simulink model "line_CF1_FS"  (R2018b)
settings: Solver=FixedStepAuto  StartTime=0.0  StopTime=inf  FixedStep=0.01  RelTol=1e-3
undefined symbols (not defined in the file or in its folder): Angular, Linear
libraries: autolibshared x10, vehdynlibsteering x10, robotlib x7, peGeneralControl x1
(part 1 of 2)
settings Model: Creator=ckreienk  LastModifiedBy=ckreienk

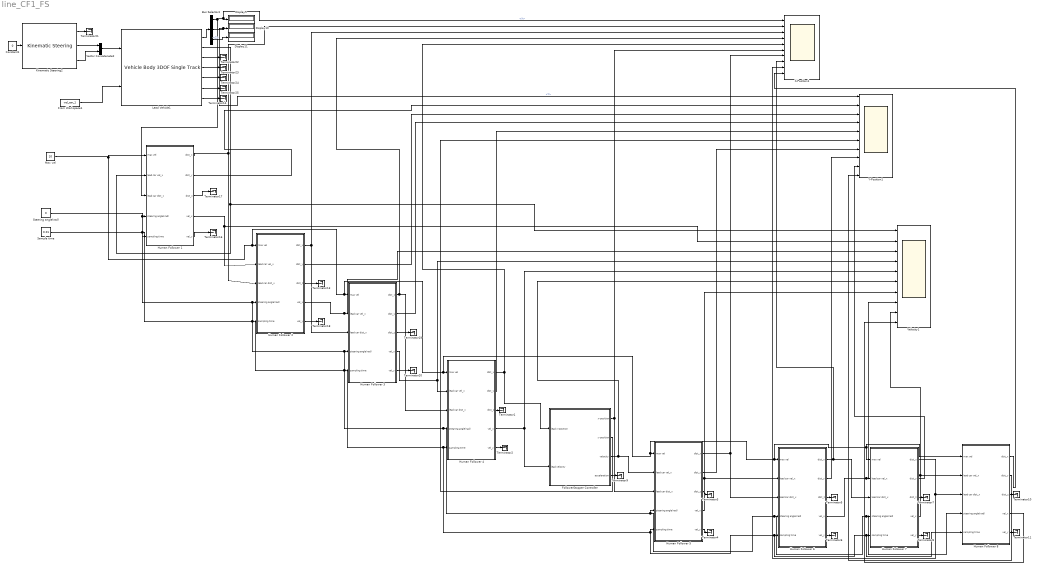
== system line_CF1_FS ==
  Bus Selector4 : BusSelector  OutputSignals=InertFrm.Geom.Disp.X,InertFrm.Geom.Disp.Y,InertFrm.Geom.Disp.Z
  Constant1 : Constant  Value=0
  Display10 : Display
  Display11 : Display
  Display9 : Display
  FollowerStopper Controller : Subsystem
  From Workspace1 : FromWorkspace  VariableName=vel_car_1  SampleTime=0.1
  Human Follower 1 : Subsystem
  Human Follower 2 : Subsystem
  Human Follower 3 : Subsystem
  Human Follower 4 : Subsystem
  Human Follower 5 : Subsystem
  Human Follower 6 : Subsystem
  Human Follower 7 : Subsystem
  Human Follower 8 : Subsystem
  Kinematic Steering2 : vehdynlibsteering/Kinematic Steering  StrgType=Rack and pinion  StrgRatioType=Constant  Loc=Front  NrmlFctr=0.01  TrckWdth=1  WhlBase=1.524  Db=0  StrgRng=1.25*pi  StrgAngBpts="[-6.2832   -5.0265   -3.7699   -2.5133   -1.2566         0    1.2566    2.5133    3.7699    5.0265    6.2832]"  StrgRatioTbl=|  StrgRatio=100  StrgArmLngth=0.1  RckCsLngth=0.5  TieRodLngth=0.248  D=0.2  PnnRadius=0.0057  PnnRadiusTbl="[0.0055    0.0055    0.0056    0.0057    0.0058    0.0057    0.0057    0.0057    0.0056    0.0055    0.0055]"  RodLngth=0.1  ParaArmLngth=0.9  aMode=2
      | [13.5000   13.3750   13.2500   13.1250   13.0000   13.0000   13.0000   13.1250   13.2500   13.3750   13.5000
      | ]
      settings: SourceProductName=Vehicle Dynamics Blockset
  Lead Vehicle1 : autolibshared/Vehicle Body 3DOF Single Track  trackMode=Dual  inputMode=External longitudinal velocity  frontSteerMode=on  rearSteerMode=off  windMode=off  muMode=off  extFMode=off  extMMode=off  aMode=2  NF=2  NR=2  m=2000  a=1.4  b=1.6  h=0.35  X_o=100  xdot_o=0  CalphaMode=off  sigmaMode=off  d=0  w=[1.4,1.4]  Cy_f=12e3  Cy_r=11e3  sigma_f=.1  sigma_r=.1  alpha_f_brk=[-.1 .1]  Cy_f_data=[-9e3 9e3]  alpha_r_brk=[-.1 .1]  Cy_r_data=[-9e3 9e3]  Y_o=0  ydot_o=0  Izz=4000  psi_o=0  r_o=0  Af=2  Cd=.3  Cl=.1  Cpm=.1  beta_w=[0:0.01:0.3]  Cs=[0:0.03:0.9]  Cym=[0:0.01:0.3]  Pabs=101325  Tair=273  g=9.81  mu=1  xdot_tol=.01  Fznom=5000  Fxtire_sat=7e4  Fytire_sat=7e4  longOff=0  latOff=0  vertOff=0
      settings: SourceProductName=Powertrain Blockset  SourceProductBaseCode=PW
  Max vel : Constant  Value=10
  Sample time : Constant  Value=0.01
  Steering angle(rad) : Constant  Value=0
  Terminator{1..11,13..14,16..25} (23 alike) : Terminator
  Vector Concatenate2 : Concatenate
  Velocity1 : Scope  NumInputPorts=10
  X-Position1 : Scope  NumInputPorts=10
  Y-Position1 : Scope  NumInputPorts=10
  wires:
  Human Follower 1/2(dist_y) -> Y-Position1/2
  Human Follower 2/5(vel_y) -> Terminator18/1
  Human Follower 1/4(vel_x) -> Human Follower 2/2(lead car vel_x), Velocity1/2
  Human Follower 3/5(vel_y) -> Terminator20/1
  Human Follower 3/4(vel_x) -> Human Follower 4/2(lead car vel_x), Velocity1/4
  Vector Concatenate2/1 -> Lead Vehicle1/1
  Lead Vehicle1/7 -> Terminator14/1
  Human Follower 1/1(dist_x) -> Human Follower 2/3(lead car dist_x), X-Position1/2
  Human Follower 2/1(dist_x) -> X-Position1/3, Human Follower 3/3(lead car dist_x)
  Sample time/1 -> Human Follower 8/5(sampling time), Human Follower 7/5(sampling time), Human Follower 6/5(sampling time), Human Follower 5/5(sampling time), Human Follower 4/5(sampling time), Human Follower 3/5(sampling time), Human Follower 2/5(sampling time), Human Follower 1/5(sampling time)
  Max vel/1 -> Human Follower 1/1(max vel), Human Follower 7/1(max vel), Human Follower 8/1(max vel), Human Follower 6/1(max vel), Human Follower 5/1(max vel), Human Follower 4/1(max vel), Human Follower 3/1(max vel), Human Follower 2/1(max vel)
  Lead Vehicle1/6 -> Terminator25/1
  Bus Selector4/1 -> Display9/1, X-Position1/1, Human Follower 1/3(lead car dist_x)  "<X>"
  Kinematic Steering2/2 -> Vector Concatenate2/1
  Lead Vehicle1/4 -> Terminator23/1
  Human Follower 1/3(dist_z) -> Terminator17/1
  Human Follower 2/4(vel_x) -> Velocity1/3, Human Follower 3/2(lead car vel_x)
  Lead Vehicle1/2 -> Human Follower 1/2(lead car vel_x), Velocity1/1
  Constant1/1 -> Kinematic Steering2/1
  Human Follower 2/3(dist_z) -> Terminator13/1
  Lead Vehicle1/1 -> Bus Selector4/1
  Lead Vehicle1/3 -> Terminator22/1
  Human Follower 3/3(dist_z) -> Terminator19/1
  From Workspace1/1 -> Lead Vehicle1/2
  Human Follower 2/2(dist_y) -> Y-Position1/3
  Human Follower 3/2(dist_y) -> Y-Position1/4
  Human Follower 3/1(dist_x) -> Human Follower 4/3(lead car dist_x), X-Position1/4
  Bus Selector4/2 -> Display10/1, Y-Position1/1  "<Y>"
  Kinematic Steering2/1 -> Terminator21/1
  Kinematic Steering2/3 -> Vector Concatenate2/2
  Bus Selector4/3 -> Display11/1  "<Z>"
  Human Follower 1/5(vel_y) -> Terminator16/1
  Lead Vehicle1/5 -> Terminator24/1
  Steering angle(rad)/1 -> Human Follower 8/4(stearing angle(rad)), Human Follower 7/4(stearing angle(rad)), Human Follower 6/4(stearing angle(rad)), Human Follower 5/4(stearing angle(rad)), Human Follower 4/4(stearing angle(rad)), Human Follower 3/4(stearing angle(rad)), Human Follower 2/4(stearing angle(rad)), Human Follower 1/4(stearing angle(rad))
  Human Follower 4/1(dist_x) -> X-Position1/5, FollowerStopper Controller/1(lead x-position)
  Human Follower 4/2(dist_y) -> Y-Position1/5
  Human Follower 4/3(dist_z) -> Terminator1/1
  Human Follower 4/5(vel_y) -> Terminator2/1
  Human Follower 4/4(vel_x) -> FollowerStopper Controller/2(lead velocity), Velocity1/5
  Human Follower 5/5(vel_y) -> Terminator4/1
  Human Follower 5/3(dist_z) -> Terminator3/1
  Human Follower 6/5(vel_y) -> Terminator6/1
  Human Follower 6/3(dist_z) -> Terminator5/1
  Human Follower 7/5(vel_y) -> Terminator8/1
  Human Follower 7/3(dist_z) -> Terminator7/1
  FollowerStopper Controller/1(x-position) -> Human Follower 5/3(lead car dist_x), X-Position1/6
  FollowerStopper Controller/2(y-position) -> Y-Position1/6
  FollowerStopper Controller/3(velocity) -> Human Follower 5/2(lead car vel_x), Velocity1/6
  FollowerStopper Controller/4(acceleration) -> Terminator9/1
  Human Follower 5/1(dist_x) -> Human Follower 6/3(lead car dist_x), X-Position1/7
  Human Follower 5/2(dist_y) -> Y-Position1/7
  Human Follower 5/4(vel_x) -> Human Follower 6/2(lead car vel_x), Velocity1/7
  Human Follower 6/1(dist_x) -> X-Position1/8, Human Follower 7/3(lead car dist_x)
  Human Follower 6/2(dist_y) -> Y-Position1/8
  Human Follower 6/4(vel_x) -> Velocity1/8, Human Follower 7/2(lead car vel_x)
  Human Follower 7/4(vel_x) -> Velocity1/9, Human Follower 8/2(lead car vel_x)
  Human Follower 7/2(dist_y) -> Y-Position1/9
  Human Follower 7/1(dist_x) -> Human Follower 8/3(lead car dist_x), X-Position1/9
  Human Follower 8/1(dist_x) -> X-Position1/10
  Human Follower 8/2(dist_y) -> Y-Position1/10
  Human Follower 8/3(dist_z) -> Terminator10/1
  Human Follower 8/5(vel_y) -> Terminator11/1
  Human Follower 8/4(vel_x) -> Velocity1/10

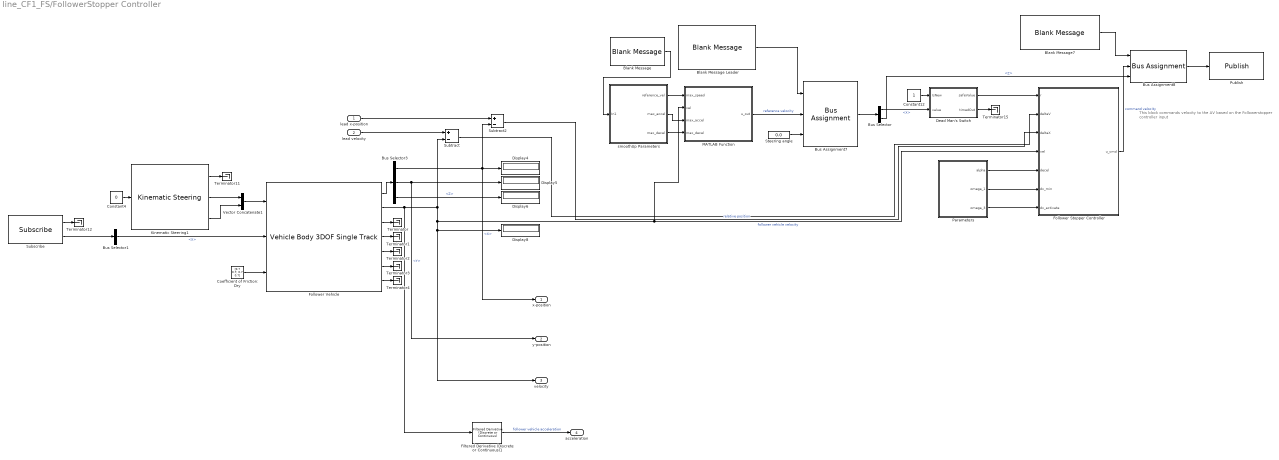
== system line_CF1_FS/FollowerStopper Controller ==
  note: This block commands velocity to the AV based
      | on the Followerstopper controller input
  lead x-position : Inport
  lead velocity : Inport  Port=2
  Blank Message : robotlib/Blank Message  messageClass=Message  entityType=geometry_msgs/Point  messageType=geometry_msgs/Point  SampleTime=inf
      settings: SourceProductBaseCode=RO
  Blank Message Leader : robotlib/Blank Message  messageClass=Message  entityType=geometry_msgs/Twist  messageType=geometry_msgs/Twist  SampleTime=inf
      settings: SourceProductBaseCode=RO
  Blank Message7 : robotlib/Blank Message  messageClass=Message  entityType=geometry_msgs/Twist  messageType=geometry_msgs/Twist  SampleTime=inf
      settings: SourceProductBaseCode=RO
  Bus Assignment7 : BusAssignment  AssignedSignals=Linear.X,Angular.Z
  Bus Assignment8 : BusAssignment  AssignedSignals=Linear.X,Angular.Z
  Bus Selector : BusSelector  OutputSignals=Linear.X,Angular.Z
  Bus Selector1 : BusSelector  OutputSignals=Linear.X
  Bus Selector3 : BusSelector  OutputSignals=InertFrm.Geom.Disp.X,InertFrm.Geom.Disp.Y,InertFrm.Geom.Disp.Z
  Coefficient of Friction: Dry : Constant  Value=[0.7 0.7; 0.7 0.7]
  Constant12 : Constant
  Constant4 : Constant  Value=0
  Dead Man's Switch : Subsystem  TreatAsAtomicUnit=on  mask{stepSize=0.05, timeout=0.2}
      mask prompts: stepSize "Simulation step size"; timeout "Timeout (in seconds)"
      mask help: Interprets whether a new message has been recently received, and if so permits the data in 'value' to be passed through. Otherwise, 0 is outputted from 'safeValue'
      mask Help: Interprets whether a new message has been recently received, and if so permits the data in 'value' to be passed through. Otherwise, 0 is outputted from 'safeValue'
  Display{4..6,8} (4 alike) : Display
  Filtered Derivative (Discrete or Continuous)1 : peGeneralControl/Filtered Derivative (Discrete or Continuous)  K=1  T=0.1  B=20  A=-20  minRatio=10  Ts=-1
  Follower Stopper Controller : Subsystem
  Follower Vehicle : autolibshared/Vehicle Body 3DOF Single Track  trackMode=Dual  inputMode=External longitudinal velocity  frontSteerMode=on  rearSteerMode=off  windMode=off  muMode=on  extFMode=off  extMMode=off  aMode=2  NF=2  NR=2  m=2000  a=1.4  b=1.6  h=0.35  X_o=50  xdot_o=0  CalphaMode=off  sigmaMode=on  d=0  w=[1.4,1.4]  Cy_f=12e3  Cy_r=11e3  sigma_f=.1  sigma_r=.1  alpha_f_brk=[-.1 .1]  Cy_f_data=[-9e3 9e3]  alpha_r_brk=[-.1 .1]  Cy_r_data=[-9e3 9e3]  Y_o=0  ydot_o=0  Izz=4000  psi_o=0  r_o=0  Af=2  Cd=.3  Cl=.1  Cpm=.1  beta_w=[0:0.01:0.3]  Cs=[0:0.03:0.9]  Cym=[0:0.01:0.3]  Pabs=101325  Tair=273  g=9.81  mu=1  xdot_tol=.01  Fznom=5000  Fxtire_sat=7e4  Fytire_sat=7e4  longOff=0  latOff=0  vertOff=0
      settings: SourceProductName=Powertrain Blockset  SourceProductBaseCode=PW
  Kinematic Steering1 : vehdynlibsteering/Kinematic Steering  StrgType=Rack and pinion  StrgRatioType=Constant  Loc=Front  NrmlFctr=0.01  TrckWdth=1  WhlBase=1.524  Db=0  StrgRng=1.25*pi  StrgAngBpts="[-6.2832   -5.0265   -3.7699   -2.5133   -1.2566         0    1.2566    2.5133    3.7699    5.0265    6.2832]"  StrgRatioTbl=|  StrgRatio=100  StrgArmLngth=0.1  RckCsLngth=0.5  TieRodLngth=0.248  D=0.2  PnnRadius=0.0057  PnnRadiusTbl="[0.0055    0.0055    0.0056    0.0057    0.0058    0.0057    0.0057    0.0057    0.0056    0.0055    0.0055]"  RodLngth=0.1  ParaArmLngth=0.9  aMode=2
      | [13.5000   13.3750   13.2500   13.1250   13.0000   13.0000   13.0000   13.1250   13.2500   13.3750   13.5000
      | ]
      settings: SourceProductName=Vehicle Dynamics Blockset
  MATLAB Function : MATLAB Function  TreatAsAtomicUnit=on
  Parameters : Subsystem
  Publish : robotlib/Publish  topicSource=Specify your own  topic=cmd_vel  messageType=geometry_msgs/Twist  messageQueueLength=1
      settings: SourceProductBaseCode=RO
  Steering angle : Constant  Value=0.0
  Subscribe : robotlib/Subscribe  topicSource=Specify your own  topic=cmd_vel  messageType=geometry_msgs/Twist  sampleTime=-1  messageQueueLength=1
      settings: SourceProductBaseCode=RO
  Subtract : Sum  Inputs=+-
  Subtract2 : Sum  Inputs=+-
  Terminator{,1..4,11..12,15} (8 alike) : Terminator
  Vector Concatenate1 : Concatenate
  smoothUp Parameters : Subsystem
  x-position : Outport
  y-position : Outport  Port=2
  velocity : Outport  Port=3
  acceleration : Outport  Port=4
  wires:
  Follower Vehicle/7 -> Terminator4/1
  MATLAB Function/1(u_out) -> Bus Assignment7/2  "reference velocity"
  Constant4/1 -> Kinematic Steering1/1
  Parameters/3(omega_3) -> Follower Stopper Controller/7(dx_activate)
  Bus Selector3/2 -> y-position/1, Display5/1  "<Y>"
  Steering angle/1 -> Bus Assignment7/3
  Follower Vehicle/5 -> Terminator2/1
  Constant12/1 -> Dead Man's Switch/1(IsNew)
  Subtract2/1 -> Follower Stopper Controller/3(deltaX)  "relative position"
  Dead Man's Switch/1(safeValue) -> Follower Stopper Controller/1(r)
  Kinematic Steering1/1 -> Terminator11/1
  Bus Selector/1 -> Dead Man's Switch/2(value)  "<X>"
  Bus Selector3/3 -> Display6/1  "<Z>"
  Dead Man's Switch/2(timedOut) -> Terminator15/1
  Subscribe/1 -> Terminator12/1
  Follower Vehicle/2 -> Filtered Derivative (Discrete or Continuous)1/1, velocity/1, Display8/1, MATLAB Function/2(vel), Follower Stopper Controller/4(vel), Subtract/2  "follower vehicle velocity"
  lead x-position/1 -> Subtract2/1
  Parameters/2(omega_1) -> Follower Stopper Controller/6(dx_min)
  Follower Stopper Controller/1(u_cmd) -> Bus Assignment8/2  "command velocity"
  Bus Selector3/1 -> x-position/1, Display4/1, Subtract2/2  "<X>"
  Blank Message/1 -> smoothUp Parameters/1(In1)
  Bus Selector1/1 -> Follower Vehicle/2  "<X>"
  Vector Concatenate1/1 -> Follower Vehicle/1
  Subtract/1 -> Follower Stopper Controller/2(deltaV)
  Blank Message Leader/1 -> Bus Assignment7/1
  Filtered Derivative (Discrete or Continuous)1/1 -> acceleration/1  "follower vehicle acceleration"
  Bus Selector/2 -> Bus Assignment8/3  "<Z>"
  Bus Assignment8/1 -> Publish/1
  Bus Assignment7/1 -> Bus Selector/1
  smoothUp Parameters/1(reference_vel) -> MATLAB Function/1(max_speed)
  Coefficient of Friction: Dry/1 -> Follower Vehicle/3
  Follower Vehicle/6 -> Terminator3/1
  Blank Message7/1 -> Bus Assignment8/1
  smoothUp Parameters/2(max_accel) -> MATLAB Function/3(max_accel)
  Follower Vehicle/1 -> Bus Selector3/1
  Follower Vehicle/3 -> Terminator/1
  Kinematic Steering1/2 -> Vector Concatenate1/1
  Kinematic Steering1/3 -> Vector Concatenate1/2
  Subscribe/2 -> Bus Selector1/1
  Parameters/1(alpha) -> Follower Stopper Controller/5(decel)
  lead velocity/1 -> Subtract/1
  smoothUp Parameters/3(max_decel) -> MATLAB Function/4(max_decel)
  Follower Vehicle/4 -> Terminator1/1

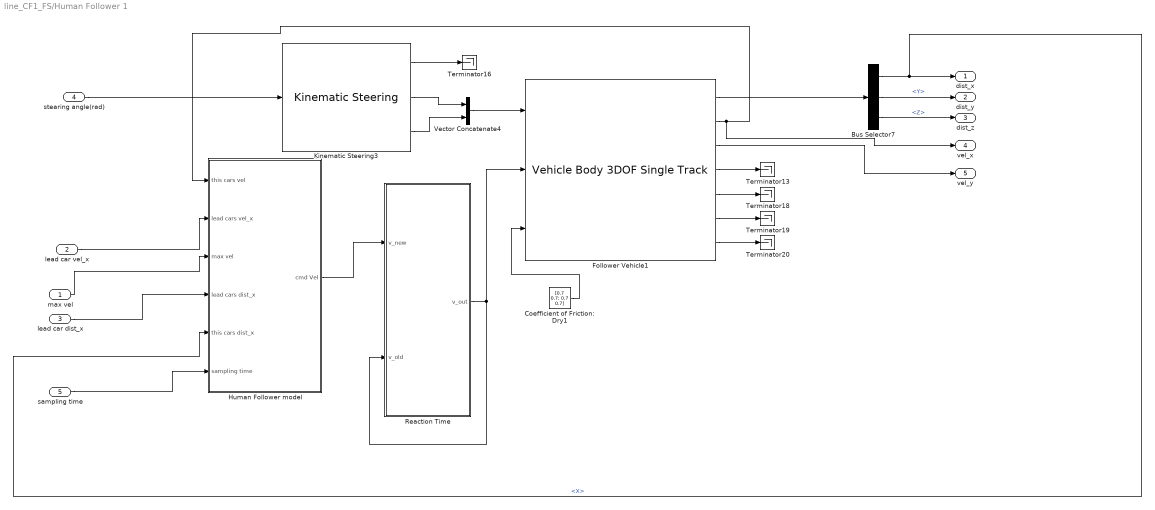
== system line_CF1_FS/Human Follower 1 ==
  max vel : Inport
  lead car vel_x : Inport  Port=2
  lead car dist_x : Inport  Port=3
  stearing angle(rad) : Inport  Port=4
  sampling time : Inport  Port=5
  Bus Selector7 : BusSelector  OutputSignals=InertFrm.Cg.Disp.X,InertFrm.Cg.Disp.Y,InertFrm.Cg.Disp.Z
  Coefficient of Friction: Dry1 : Constant  Value=[0.7 0.7; 0.7 0.7]
  Follower Vehicle1 : autolibshared/Vehicle Body 3DOF Single Track  trackMode=Dual  inputMode=External longitudinal velocity  frontSteerMode=on  rearSteerMode=off  windMode=off  muMode=on  extFMode=off  extMMode=off  aMode=2  NF=2  NR=2  m=2000  a=1.4  b=1.6  h=0.35  X_o=90  xdot_o=0  CalphaMode=off  sigmaMode=on  d=0  w=[1.4,1.4]  Cy_f=12e3  Cy_r=11e3  sigma_f=.1  sigma_r=.1  alpha_f_brk=[-.1 .1]  Cy_f_data=[-9e3 9e3]  alpha_r_brk=[-.1 .1]  Cy_r_data=[-9e3 9e3]  Y_o=0  ydot_o=0  Izz=4000  psi_o=0  r_o=0  Af=2  Cd=.3  Cl=.1  Cpm=.1  beta_w=[0:0.01:0.3]  Cs=[0:0.03:0.9]  Cym=[0:0.01:0.3]  Pabs=101325  Tair=273  g=9.81  mu=1  xdot_tol=.01  Fznom=5000  Fxtire_sat=7e4  Fytire_sat=7e4  longOff=0  latOff=0  vertOff=0
      settings: SourceProductName=Powertrain Blockset  SourceProductBaseCode=PW
  Human Follower model : Subsystem
  Kinematic Steering3 : vehdynlibsteering/Kinematic Steering  StrgType=Rack and pinion  StrgRatioType=Constant  Loc=Front  NrmlFctr=0.01  TrckWdth=1  WhlBase=1.524  Db=0  StrgRng=1.25*pi  StrgAngBpts="[-6.2832   -5.0265   -3.7699   -2.5133   -1.2566         0    1.2566    2.5133    3.7699    5.0265    6.2832]"  StrgRatioTbl=|  StrgRatio=100  StrgArmLngth=0.1  RckCsLngth=0.5  TieRodLngth=0.248  D=0.2  PnnRadius=0.0057  PnnRadiusTbl="[0.0055    0.0055    0.0056    0.0057    0.0058    0.0057    0.0057    0.0057    0.0056    0.0055    0.0055]"  RodLngth=0.1  ParaArmLngth=0.9  aMode=2
      | [13.5000   13.3750   13.2500   13.1250   13.0000   13.0000   13.0000   13.1250   13.2500   13.3750   13.5000
      | ]
      settings: SourceProductName=Vehicle Dynamics Blockset
  Reaction Time : Subsystem
  Terminator{13,16,18..20} (5 alike) : Terminator
  Vector Concatenate4 : Concatenate
  dist_x : Outport
  dist_y : Outport  Port=2
  dist_z : Outport  Port=3
  vel_x : Outport  Port=4
  vel_y : Outport  Port=5
  wires:
  Bus Selector7/3 -> dist_z/1  "<Z>"
  Follower Vehicle1/5 -> Terminator18/1
  max vel/1 -> Human Follower model/3(max vel)
  Follower Vehicle1/6 -> Terminator19/1
  Bus Selector7/1 -> dist_x/1, Human Follower model/5(this cars dist_x)  "<X>"
  Follower Vehicle1/4 -> Terminator13/1
  Follower Vehicle1/3 -> vel_y/1
  lead car vel_x/1 -> Human Follower model/2(lead cars vel_x)
  Follower Vehicle1/7 -> Terminator20/1
  Vector Concatenate4/1 -> Follower Vehicle1/1
  Follower Vehicle1/1 -> Bus Selector7/1
  Kinematic Steering3/1 -> Terminator16/1
  lead car dist_x/1 -> Human Follower model/4(lead cars dist_x)
  Bus Selector7/2 -> dist_y/1  "<Y>"
  Kinematic Steering3/2 -> Vector Concatenate4/1
  stearing angle(rad)/1 -> Kinematic Steering3/1
  Kinematic Steering3/3 -> Vector Concatenate4/2
  Follower Vehicle1/2 -> Human Follower model/1(this cars vel), vel_x/1
  Coefficient of Friction: Dry1/1 -> Follower Vehicle1/3
  sampling time/1 -> Human Follower model/6(sampling time)
  Reaction Time/1(v_out) -> Follower Vehicle1/2, Reaction Time/2(v_old)
  Human Follower model/1(cmd Vel) -> Reaction Time/1(v_new)

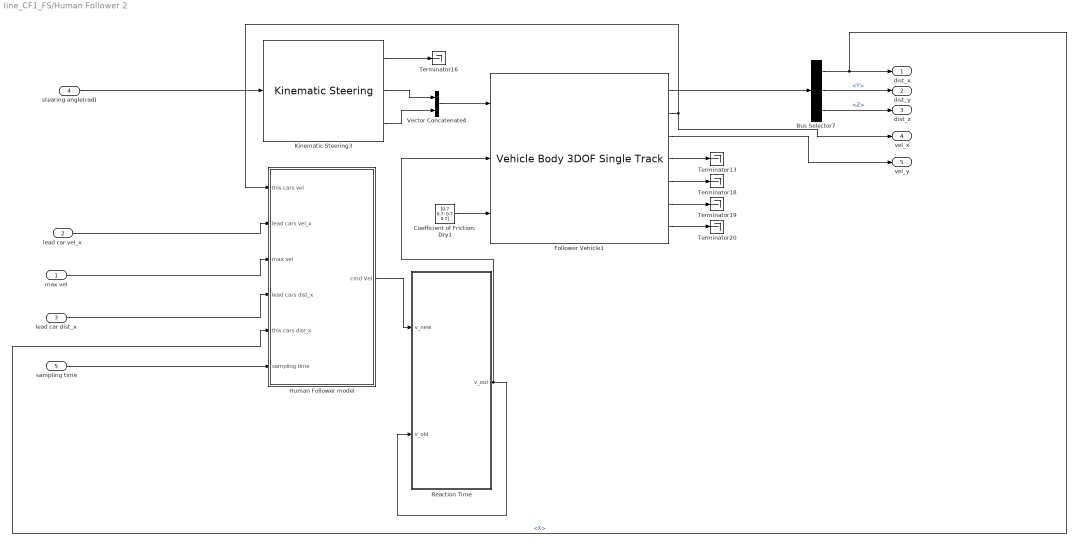
== system line_CF1_FS/Human Follower 2 ==
  max vel : Inport
  lead car vel_x : Inport  Port=2
  lead car dist_x : Inport  Port=3
  stearing angle(rad) : Inport  Port=4
  sampling time : Inport  Port=5
  Bus Selector7 : BusSelector  OutputSignals=InertFrm.Cg.Disp.X,InertFrm.Cg.Disp.Y,InertFrm.Cg.Disp.Z
  Coefficient of Friction: Dry1 : Constant  Value=[0.7 0.7; 0.7 0.7]
  Follower Vehicle1 : autolibshared/Vehicle Body 3DOF Single Track  trackMode=Dual  inputMode=External longitudinal velocity  frontSteerMode=on  rearSteerMode=off  windMode=off  muMode=on  extFMode=off  extMMode=off  aMode=2  NF=2  NR=2  m=2000  a=1.4  b=1.6  h=0.35  X_o=80  xdot_o=0  CalphaMode=off  sigmaMode=on  d=0  w=[1.4,1.4]  Cy_f=12e3  Cy_r=11e3  sigma_f=.1  sigma_r=.1  alpha_f_brk=[-.1 .1]  Cy_f_data=[-9e3 9e3]  alpha_r_brk=[-.1 .1]  Cy_r_data=[-9e3 9e3]  Y_o=0  ydot_o=0  Izz=4000  psi_o=0  r_o=0  Af=2  Cd=.3  Cl=.1  Cpm=.1  beta_w=[0:0.01:0.3]  Cs=[0:0.03:0.9]  Cym=[0:0.01:0.3]  Pabs=101325  Tair=273  g=9.81  mu=1  xdot_tol=.01  Fznom=5000  Fxtire_sat=7e4  Fytire_sat=7e4  longOff=0  latOff=0  vertOff=0
      settings: SourceProductName=Powertrain Blockset  SourceProductBaseCode=PW
  Human Follower model : Subsystem
  Kinematic Steering3 : vehdynlibsteering/Kinematic Steering  StrgType=Rack and pinion  StrgRatioType=Constant  Loc=Front  NrmlFctr=0.01  TrckWdth=1  WhlBase=1.524  Db=0  StrgRng=1.25*pi  StrgAngBpts="[-6.2832   -5.0265   -3.7699   -2.5133   -1.2566         0    1.2566    2.5133    3.7699    5.0265    6.2832]"  StrgRatioTbl=|  StrgRatio=100  StrgArmLngth=0.1  RckCsLngth=0.5  TieRodLngth=0.248  D=0.2  PnnRadius=0.0057  PnnRadiusTbl="[0.0055    0.0055    0.0056    0.0057    0.0058    0.0057    0.0057    0.0057    0.0056    0.0055    0.0055]"  RodLngth=0.1  ParaArmLngth=0.9  aMode=2
      | [13.5000   13.3750   13.2500   13.1250   13.0000   13.0000   13.0000   13.1250   13.2500   13.3750   13.5000
      | ]
      settings: SourceProductName=Vehicle Dynamics Blockset
  Reaction Time : Subsystem
  Terminator{13,16,18..20} (5 alike) : Terminator
  Vector Concatenate4 : Concatenate
  dist_x : Outport
  dist_y : Outport  Port=2
  dist_z : Outport  Port=3
  vel_x : Outport  Port=4
  vel_y : Outport  Port=5
  wires:
  Bus Selector7/3 -> dist_z/1  "<Z>"
  Follower Vehicle1/5 -> Terminator18/1
  max vel/1 -> Human Follower model/3(max vel)
  Follower Vehicle1/6 -> Terminator19/1
  Bus Selector7/1 -> dist_x/1, Human Follower model/5(this cars dist_x)  "<X>"
  Follower Vehicle1/4 -> Terminator13/1
  Follower Vehicle1/3 -> vel_y/1
  lead car vel_x/1 -> Human Follower model/2(lead cars vel_x)
  Follower Vehicle1/7 -> Terminator20/1
  Vector Concatenate4/1 -> Follower Vehicle1/1
  Follower Vehicle1/1 -> Bus Selector7/1
  Kinematic Steering3/1 -> Terminator16/1
  lead car dist_x/1 -> Human Follower model/4(lead cars dist_x)
  Bus Selector7/2 -> dist_y/1  "<Y>"
  sampling time/1 -> Human Follower model/6(sampling time)
  Kinematic Steering3/2 -> Vector Concatenate4/1
  stearing angle(rad)/1 -> Kinematic Steering3/1
  Kinematic Steering3/3 -> Vector Concatenate4/2
  Follower Vehicle1/2 -> Human Follower model/1(this cars vel), vel_x/1
  Coefficient of Friction: Dry1/1 -> Follower Vehicle1/3
  Reaction Time/1(v_out) -> Follower Vehicle1/2, Reaction Time/2(v_old)
  Human Follower model/1(cmd Vel) -> Reaction Time/1(v_new)

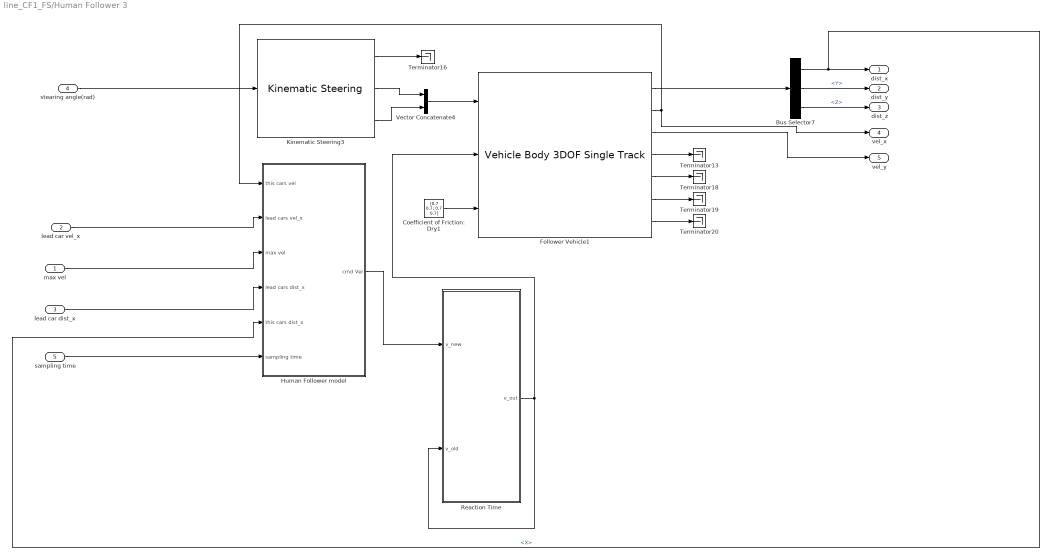
== system line_CF1_FS/Human Follower 3 ==
  max vel : Inport
  lead car vel_x : Inport  Port=2
  lead car dist_x : Inport  Port=3
  stearing angle(rad) : Inport  Port=4
  sampling time : Inport  Port=5
  Bus Selector7 : BusSelector  OutputSignals=InertFrm.Cg.Disp.X,InertFrm.Cg.Disp.Y,InertFrm.Cg.Disp.Z
  Coefficient of Friction: Dry1 : Constant  Value=[0.7 0.7; 0.7 0.7]
  Follower Vehicle1 : autolibshared/Vehicle Body 3DOF Single Track  trackMode=Dual  inputMode=External longitudinal velocity  frontSteerMode=on  rearSteerMode=off  windMode=off  muMode=on  extFMode=off  extMMode=off  aMode=2  NF=2  NR=2  m=2000  a=1.4  b=1.6  h=0.35  X_o=70  xdot_o=0  CalphaMode=off  sigmaMode=on  d=0  w=[1.4,1.4]  Cy_f=12e3  Cy_r=11e3  sigma_f=.1  sigma_r=.1  alpha_f_brk=[-.1 .1]  Cy_f_data=[-9e3 9e3]  alpha_r_brk=[-.1 .1]  Cy_r_data=[-9e3 9e3]  Y_o=0  ydot_o=0  Izz=4000  psi_o=0  r_o=0  Af=2  Cd=.3  Cl=.1  Cpm=.1  beta_w=[0:0.01:0.3]  Cs=[0:0.03:0.9]  Cym=[0:0.01:0.3]  Pabs=101325  Tair=273  g=9.81  mu=1  xdot_tol=.01  Fznom=5000  Fxtire_sat=7e4  Fytire_sat=7e4  longOff=0  latOff=0  vertOff=0
      settings: SourceProductName=Powertrain Blockset  SourceProductBaseCode=PW
  Human Follower model : Subsystem
  Kinematic Steering3 : vehdynlibsteering/Kinematic Steering  StrgType=Rack and pinion  StrgRatioType=Constant  Loc=Front  NrmlFctr=0.01  TrckWdth=1  WhlBase=1.524  Db=0  StrgRng=1.25*pi  StrgAngBpts="[-6.2832   -5.0265   -3.7699   -2.5133   -1.2566         0    1.2566    2.5133    3.7699    5.0265    6.2832]"  StrgRatioTbl=|  StrgRatio=100  StrgArmLngth=0.1  RckCsLngth=0.5  TieRodLngth=0.248  D=0.2  PnnRadius=0.0057  PnnRadiusTbl="[0.0055    0.0055    0.0056    0.0057    0.0058    0.0057    0.0057    0.0057    0.0056    0.0055    0.0055]"  RodLngth=0.1  ParaArmLngth=0.9  aMode=2
      | [13.5000   13.3750   13.2500   13.1250   13.0000   13.0000   13.0000   13.1250   13.2500   13.3750   13.5000
      | ]
      settings: SourceProductName=Vehicle Dynamics Blockset
  Reaction Time : Subsystem
  Terminator{13,16,18..20} (5 alike) : Terminator
  Vector Concatenate4 : Concatenate
  dist_x : Outport
  dist_y : Outport  Port=2
  dist_z : Outport  Port=3
  vel_x : Outport  Port=4
  vel_y : Outport  Port=5
  wires:
  Bus Selector7/3 -> dist_z/1  "<Z>"
  Follower Vehicle1/5 -> Terminator18/1
  max vel/1 -> Human Follower model/3(max vel)
  Follower Vehicle1/6 -> Terminator19/1
  Bus Selector7/1 -> dist_x/1, Human Follower model/5(this cars dist_x)  "<X>"
  Follower Vehicle1/4 -> Terminator13/1
  Follower Vehicle1/3 -> vel_y/1
  lead car vel_x/1 -> Human Follower model/2(lead cars vel_x)
  Follower Vehicle1/7 -> Terminator20/1
  Vector Concatenate4/1 -> Follower Vehicle1/1
  Follower Vehicle1/1 -> Bus Selector7/1
  Kinematic Steering3/1 -> Terminator16/1
  lead car dist_x/1 -> Human Follower model/4(lead cars dist_x)
  Bus Selector7/2 -> dist_y/1  "<Y>"
  sampling time/1 -> Human Follower model/6(sampling time)
  Kinematic Steering3/2 -> Vector Concatenate4/1
  stearing angle(rad)/1 -> Kinematic Steering3/1
  Kinematic Steering3/3 -> Vector Concatenate4/2
  Follower Vehicle1/2 -> Human Follower model/1(this cars vel), vel_x/1
  Coefficient of Friction: Dry1/1 -> Follower Vehicle1/3
  Reaction Time/1(v_out) -> Follower Vehicle1/2, Reaction Time/2(v_old)
  Human Follower model/1(cmd Vel) -> Reaction Time/1(v_new)

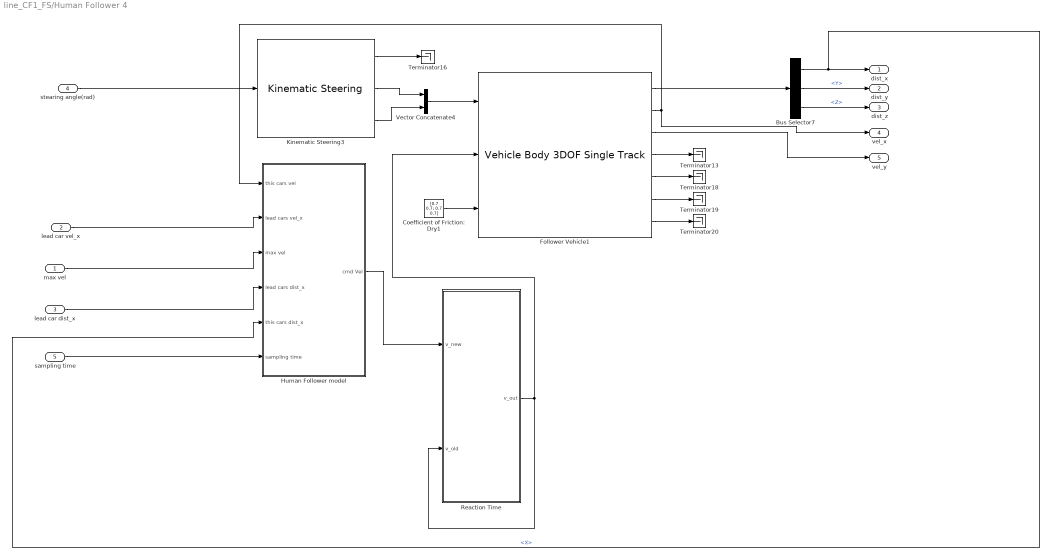
== system line_CF1_FS/Human Follower 4 ==
  max vel : Inport
  lead car vel_x : Inport  Port=2
  lead car dist_x : Inport  Port=3
  stearing angle(rad) : Inport  Port=4
  sampling time : Inport  Port=5
  Bus Selector7 : BusSelector  OutputSignals=InertFrm.Cg.Disp.X,InertFrm.Cg.Disp.Y,InertFrm.Cg.Disp.Z
  Coefficient of Friction: Dry1 : Constant  Value=[0.7 0.7; 0.7 0.7]
  Follower Vehicle1 : autolibshared/Vehicle Body 3DOF Single Track  trackMode=Dual  inputMode=External longitudinal velocity  frontSteerMode=on  rearSteerMode=off  windMode=off  muMode=on  extFMode=off  extMMode=off  aMode=2  NF=2  NR=2  m=2000  a=1.4  b=1.6  h=0.35  X_o=60  xdot_o=0  CalphaMode=off  sigmaMode=on  d=0  w=[1.4,1.4]  Cy_f=12e3  Cy_r=11e3  sigma_f=.1  sigma_r=.1  alpha_f_brk=[-.1 .1]  Cy_f_data=[-9e3 9e3]  alpha_r_brk=[-.1 .1]  Cy_r_data=[-9e3 9e3]  Y_o=0  ydot_o=0  Izz=4000  psi_o=0  r_o=0  Af=2  Cd=.3  Cl=.1  Cpm=.1  beta_w=[0:0.01:0.3]  Cs=[0:0.03:0.9]  Cym=[0:0.01:0.3]  Pabs=101325  Tair=273  g=9.81  mu=1  xdot_tol=.01  Fznom=5000  Fxtire_sat=7e4  Fytire_sat=7e4  longOff=0  latOff=0  vertOff=0
      settings: SourceProductName=Powertrain Blockset  SourceProductBaseCode=PW
  Human Follower model : Subsystem
  Kinematic Steering3 : vehdynlibsteering/Kinematic Steering  StrgType=Rack and pinion  StrgRatioType=Constant  Loc=Front  NrmlFctr=0.01  TrckWdth=1  WhlBase=1.524  Db=0  StrgRng=1.25*pi  StrgAngBpts="[-6.2832   -5.0265   -3.7699   -2.5133   -1.2566         0    1.2566    2.5133    3.7699    5.0265    6.2832]"  StrgRatioTbl=|  StrgRatio=100  StrgArmLngth=0.1  RckCsLngth=0.5  TieRodLngth=0.248  D=0.2  PnnRadius=0.0057  PnnRadiusTbl="[0.0055    0.0055    0.0056    0.0057    0.0058    0.0057    0.0057    0.0057    0.0056    0.0055    0.0055]"  RodLngth=0.1  ParaArmLngth=0.9  aMode=2
      | [13.5000   13.3750   13.2500   13.1250   13.0000   13.0000   13.0000   13.1250   13.2500   13.3750   13.5000
      | ]
      settings: SourceProductName=Vehicle Dynamics Blockset
  Reaction Time : Subsystem
  Terminator{13,16,18..20} (5 alike) : Terminator
  Vector Concatenate4 : Concatenate
  dist_x : Outport
  dist_y : Outport  Port=2
  dist_z : Outport  Port=3
  vel_x : Outport  Port=4
  vel_y : Outport  Port=5
  wires:
  Bus Selector7/3 -> dist_z/1  "<Z>"
  Follower Vehicle1/5 -> Terminator18/1
  max vel/1 -> Human Follower model/3(max vel)
  Follower Vehicle1/6 -> Terminator19/1
  Bus Selector7/1 -> dist_x/1, Human Follower model/5(this cars dist_x)  "<X>"
  Follower Vehicle1/4 -> Terminator13/1
  Follower Vehicle1/3 -> vel_y/1
  lead car vel_x/1 -> Human Follower model/2(lead cars vel_x)
  Follower Vehicle1/7 -> Terminator20/1
  Vector Concatenate4/1 -> Follower Vehicle1/1
  Follower Vehicle1/1 -> Bus Selector7/1
  Kinematic Steering3/1 -> Terminator16/1
  lead car dist_x/1 -> Human Follower model/4(lead cars dist_x)
  Bus Selector7/2 -> dist_y/1  "<Y>"
  sampling time/1 -> Human Follower model/6(sampling time)
  Kinematic Steering3/2 -> Vector Concatenate4/1
  stearing angle(rad)/1 -> Kinematic Steering3/1
  Kinematic Steering3/3 -> Vector Concatenate4/2
  Follower Vehicle1/2 -> Human Follower model/1(this cars vel), vel_x/1
  Coefficient of Friction: Dry1/1 -> Follower Vehicle1/3
  Reaction Time/1(v_out) -> Follower Vehicle1/2, Reaction Time/2(v_old)
  Human Follower model/1(cmd Vel) -> Reaction Time/1(v_new)

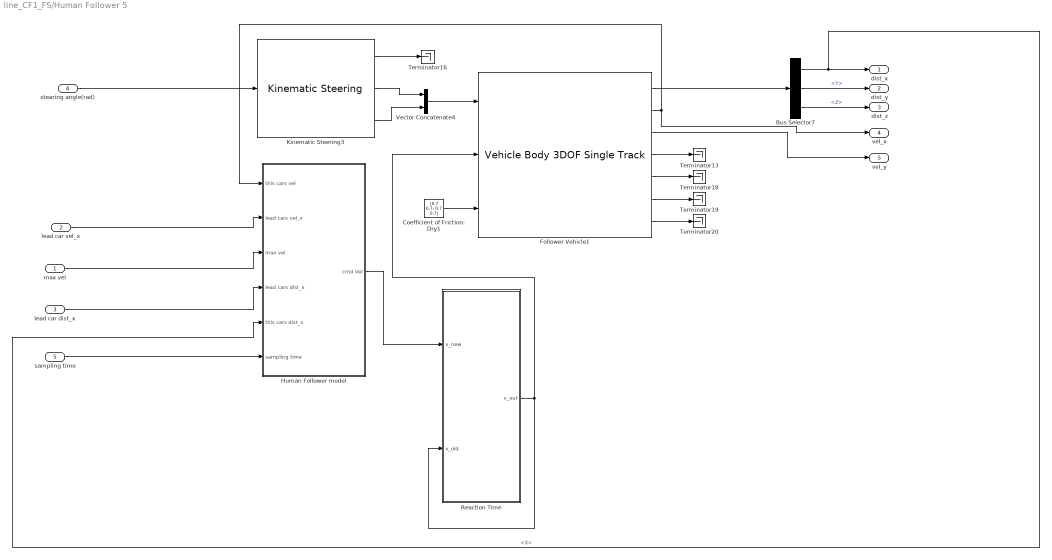
== system line_CF1_FS/Human Follower 5 ==
  max vel : Inport
  lead car vel_x : Inport  Port=2
  lead car dist_x : Inport  Port=3
  stearing angle(rad) : Inport  Port=4
  sampling time : Inport  Port=5
  Bus Selector7 : BusSelector  OutputSignals=InertFrm.Cg.Disp.X,InertFrm.Cg.Disp.Y,InertFrm.Cg.Disp.Z
  Coefficient of Friction: Dry1 : Constant  Value=[0.7 0.7; 0.7 0.7]
  Follower Vehicle1 : autolibshared/Vehicle Body 3DOF Single Track  trackMode=Dual  inputMode=External longitudinal velocity  frontSteerMode=on  rearSteerMode=off  windMode=off  muMode=on  extFMode=off  extMMode=off  aMode=2  NF=2  NR=2  m=2000  a=1.4  b=1.6  h=0.35  X_o=40  xdot_o=0  CalphaMode=off  sigmaMode=on  d=0  w=[1.4,1.4]  Cy_f=12e3  Cy_r=11e3  sigma_f=.1  sigma_r=.1  alpha_f_brk=[-.1 .1]  Cy_f_data=[-9e3 9e3]  alpha_r_brk=[-.1 .1]  Cy_r_data=[-9e3 9e3]  Y_o=0  ydot_o=0  Izz=4000  psi_o=0  r_o=0  Af=2  Cd=.3  Cl=.1  Cpm=.1  beta_w=[0:0.01:0.3]  Cs=[0:0.03:0.9]  Cym=[0:0.01:0.3]  Pabs=101325  Tair=273  g=9.81  mu=1  xdot_tol=.01  Fznom=5000  Fxtire_sat=7e4  Fytire_sat=7e4  longOff=0  latOff=0  vertOff=0
      settings: SourceProductName=Powertrain Blockset  SourceProductBaseCode=PW
  Human Follower model : Subsystem
  Kinematic Steering3 : vehdynlibsteering/Kinematic Steering  StrgType=Rack and pinion  StrgRatioType=Constant  Loc=Front  NrmlFctr=0.01  TrckWdth=1  WhlBase=1.524  Db=0  StrgRng=1.25*pi  StrgAngBpts="[-6.2832   -5.0265   -3.7699   -2.5133   -1.2566         0    1.2566    2.5133    3.7699    5.0265    6.2832]"  StrgRatioTbl=|  StrgRatio=100  StrgArmLngth=0.1  RckCsLngth=0.5  TieRodLngth=0.248  D=0.2  PnnRadius=0.0057  PnnRadiusTbl="[0.0055    0.0055    0.0056    0.0057    0.0058    0.0057    0.0057    0.0057    0.0056    0.0055    0.0055]"  RodLngth=0.1  ParaArmLngth=0.9  aMode=2
      | [13.5000   13.3750   13.2500   13.1250   13.0000   13.0000   13.0000   13.1250   13.2500   13.3750   13.5000
      | ]
      settings: SourceProductName=Vehicle Dynamics Blockset
  Reaction Time : Subsystem
  Terminator{13,16,18..20} (5 alike) : Terminator
  Vector Concatenate4 : Concatenate
  dist_x : Outport
  dist_y : Outport  Port=2
  dist_z : Outport  Port=3
  vel_x : Outport  Port=4
  vel_y : Outport  Port=5
  wires:
  Bus Selector7/3 -> dist_z/1  "<Z>"
  Follower Vehicle1/5 -> Terminator18/1
  max vel/1 -> Human Follower model/3(max vel)
  Follower Vehicle1/6 -> Terminator19/1
  Bus Selector7/1 -> dist_x/1, Human Follower model/5(this cars dist_x)  "<X>"
  Follower Vehicle1/4 -> Terminator13/1
  Follower Vehicle1/3 -> vel_y/1
  lead car vel_x/1 -> Human Follower model/2(lead cars vel_x)
  Follower Vehicle1/7 -> Terminator20/1
  Vector Concatenate4/1 -> Follower Vehicle1/1
  Follower Vehicle1/1 -> Bus Selector7/1
  Kinematic Steering3/1 -> Terminator16/1
  lead car dist_x/1 -> Human Follower model/4(lead cars dist_x)
  Bus Selector7/2 -> dist_y/1  "<Y>"
  sampling time/1 -> Human Follower model/6(sampling time)
  Kinematic Steering3/2 -> Vector Concatenate4/1
  stearing angle(rad)/1 -> Kinematic Steering3/1
  Kinematic Steering3/3 -> Vector Concatenate4/2
  Follower Vehicle1/2 -> Human Follower model/1(this cars vel), vel_x/1
  Coefficient of Friction: Dry1/1 -> Follower Vehicle1/3
  Reaction Time/1(v_out) -> Follower Vehicle1/2, Reaction Time/2(v_old)
  Human Follower model/1(cmd Vel) -> Reaction Time/1(v_new)

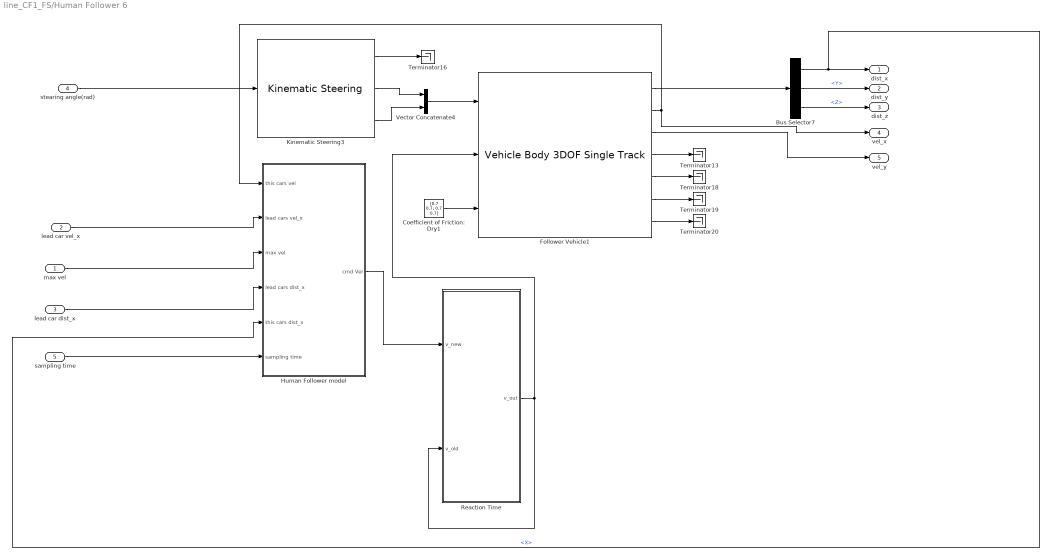
== system line_CF1_FS/Human Follower 6 ==
  max vel : Inport
  lead car vel_x : Inport  Port=2
  lead car dist_x : Inport  Port=3
  stearing angle(rad) : Inport  Port=4
  sampling time : Inport  Port=5
  Bus Selector7 : BusSelector  OutputSignals=InertFrm.Cg.Disp.X,InertFrm.Cg.Disp.Y,InertFrm.Cg.Disp.Z
  Coefficient of Friction: Dry1 : Constant  Value=[0.7 0.7; 0.7 0.7]
  Follower Vehicle1 : autolibshared/Vehicle Body 3DOF Single Track  trackMode=Dual  inputMode=External longitudinal velocity  frontSteerMode=on  rearSteerMode=off  windMode=off  muMode=on  extFMode=off  extMMode=off  aMode=2  NF=2  NR=2  m=2000  a=1.4  b=1.6  h=0.35  X_o=30  xdot_o=0  CalphaMode=off  sigmaMode=on  d=0  w=[1.4,1.4]  Cy_f=12e3  Cy_r=11e3  sigma_f=.1  sigma_r=.1  alpha_f_brk=[-.1 .1]  Cy_f_data=[-9e3 9e3]  alpha_r_brk=[-.1 .1]  Cy_r_data=[-9e3 9e3]  Y_o=0  ydot_o=0  Izz=4000  psi_o=0  r_o=0  Af=2  Cd=.3  Cl=.1  Cpm=.1  beta_w=[0:0.01:0.3]  Cs=[0:0.03:0.9]  Cym=[0:0.01:0.3]  Pabs=101325  Tair=273  g=9.81  mu=1  xdot_tol=.01  Fznom=5000  Fxtire_sat=7e4  Fytire_sat=7e4  longOff=0  latOff=0  vertOff=0
      settings: SourceProductName=Powertrain Blockset  SourceProductBaseCode=PW
  Human Follower model : Subsystem
  Kinematic Steering3 : vehdynlibsteering/Kinematic Steering  StrgType=Rack and pinion  StrgRatioType=Constant  Loc=Front  NrmlFctr=0.01  TrckWdth=1  WhlBase=1.524  Db=0  StrgRng=1.25*pi  StrgAngBpts="[-6.2832   -5.0265   -3.7699   -2.5133   -1.2566         0    1.2566    2.5133    3.7699    5.0265    6.2832]"  StrgRatioTbl=|  StrgRatio=100  StrgArmLngth=0.1  RckCsLngth=0.5  TieRodLngth=0.248  D=0.2  PnnRadius=0.0057  PnnRadiusTbl="[0.0055    0.0055    0.0056    0.0057    0.0058    0.0057    0.0057    0.0057    0.0056    0.0055    0.0055]"  RodLngth=0.1  ParaArmLngth=0.9  aMode=2
      | [13.5000   13.3750   13.2500   13.1250   13.0000   13.0000   13.0000   13.1250   13.2500   13.3750   13.5000
      | ]
      settings: SourceProductName=Vehicle Dynamics Blockset
  Reaction Time : Subsystem
  Terminator{13,16,18..20} (5 alike) : Terminator
  Vector Concatenate4 : Concatenate
  dist_x : Outport
  dist_y : Outport  Port=2
  dist_z : Outport  Port=3
  vel_x : Outport  Port=4
  vel_y : Outport  Port=5
  wires:
  Bus Selector7/3 -> dist_z/1  "<Z>"
  Follower Vehicle1/5 -> Terminator18/1
  max vel/1 -> Human Follower model/3(max vel)
  Follower Vehicle1/6 -> Terminator19/1
  Bus Selector7/1 -> dist_x/1, Human Follower model/5(this cars dist_x)  "<X>"
  Follower Vehicle1/4 -> Terminator13/1
  Follower Vehicle1/3 -> vel_y/1
  lead car vel_x/1 -> Human Follower model/2(lead cars vel_x)
  Follower Vehicle1/7 -> Terminator20/1
  Vector Concatenate4/1 -> Follower Vehicle1/1
  Follower Vehicle1/1 -> Bus Selector7/1
  Kinematic Steering3/1 -> Terminator16/1
  lead car dist_x/1 -> Human Follower model/4(lead cars dist_x)
  Bus Selector7/2 -> dist_y/1  "<Y>"
  sampling time/1 -> Human Follower model/6(sampling time)
  Kinematic Steering3/2 -> Vector Concatenate4/1
  stearing angle(rad)/1 -> Kinematic Steering3/1
  Kinematic Steering3/3 -> Vector Concatenate4/2
  Follower Vehicle1/2 -> Human Follower model/1(this cars vel), vel_x/1
  Coefficient of Friction: Dry1/1 -> Follower Vehicle1/3
  Reaction Time/1(v_out) -> Follower Vehicle1/2, Reaction Time/2(v_old)
  Human Follower model/1(cmd Vel) -> Reaction Time/1(v_new)

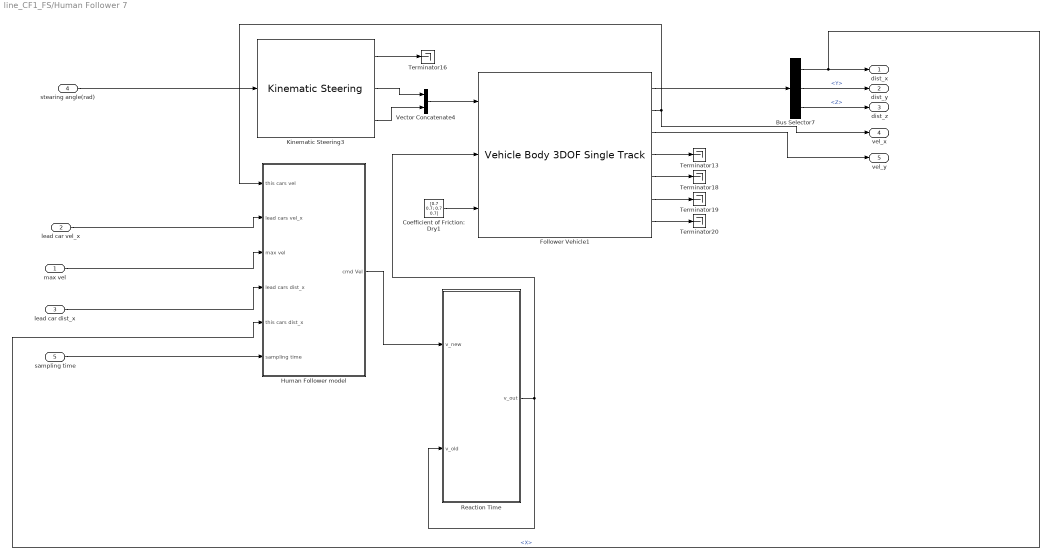
== system line_CF1_FS/Human Follower 7 ==
  max vel : Inport
  lead car vel_x : Inport  Port=2
  lead car dist_x : Inport  Port=3
  stearing angle(rad) : Inport  Port=4
  sampling time : Inport  Port=5
  Bus Selector7 : BusSelector  OutputSignals=InertFrm.Cg.Disp.X,InertFrm.Cg.Disp.Y,InertFrm.Cg.Disp.Z
  Coefficient of Friction: Dry1 : Constant  Value=[0.7 0.7; 0.7 0.7]
  Follower Vehicle1 : autolibshared/Vehicle Body 3DOF Single Track  trackMode=Dual  inputMode=External longitudinal velocity  frontSteerMode=on  rearSteerMode=off  windMode=off  muMode=on  extFMode=off  extMMode=off  aMode=2  NF=2  NR=2  m=2000  a=1.4  b=1.6  h=0.35  X_o=20  xdot_o=0  CalphaMode=off  sigmaMode=on  d=0  w=[1.4,1.4]  Cy_f=12e3  Cy_r=11e3  sigma_f=.1  sigma_r=.1  alpha_f_brk=[-.1 .1]  Cy_f_data=[-9e3 9e3]  alpha_r_brk=[-.1 .1]  Cy_r_data=[-9e3 9e3]  Y_o=0  ydot_o=0  Izz=4000  psi_o=0  r_o=0  Af=2  Cd=.3  Cl=.1  Cpm=.1  beta_w=[0:0.01:0.3]  Cs=[0:0.03:0.9]  Cym=[0:0.01:0.3]  Pabs=101325  Tair=273  g=9.81  mu=1  xdot_tol=.01  Fznom=5000  Fxtire_sat=7e4  Fytire_sat=7e4  longOff=0  latOff=0  vertOff=0
      settings: SourceProductName=Powertrain Blockset  SourceProductBaseCode=PW
  Human Follower model : Subsystem
  Kinematic Steering3 : vehdynlibsteering/Kinematic Steering  StrgType=Rack and pinion  StrgRatioType=Constant  Loc=Front  NrmlFctr=0.01  TrckWdth=1  WhlBase=1.524  Db=0  StrgRng=1.25*pi  StrgAngBpts="[-6.2832   -5.0265   -3.7699   -2.5133   -1.2566         0    1.2566    2.5133    3.7699    5.0265    6.2832]"  StrgRatioTbl=|  StrgRatio=100  StrgArmLngth=0.1  RckCsLngth=0.5  TieRodLngth=0.248  D=0.2  PnnRadius=0.0057  PnnRadiusTbl="[0.0055    0.0055    0.0056    0.0057    0.0058    0.0057    0.0057    0.0057    0.0056    0.0055    0.0055]"  RodLngth=0.1  ParaArmLngth=0.9  aMode=2
      | [13.5000   13.3750   13.2500   13.1250   13.0000   13.0000   13.0000   13.1250   13.2500   13.3750   13.5000
      | ]
      settings: SourceProductName=Vehicle Dynamics Blockset
  Reaction Time : Subsystem
  Terminator{13,16,18..20} (5 alike) : Terminator
  Vector Concatenate4 : Concatenate
  dist_x : Outport
  dist_y : Outport  Port=2
  dist_z : Outport  Port=3
  vel_x : Outport  Port=4
  vel_y : Outport  Port=5
  wires:
  Bus Selector7/3 -> dist_z/1  "<Z>"
  Follower Vehicle1/5 -> Terminator18/1
  max vel/1 -> Human Follower model/3(max vel)
  Follower Vehicle1/6 -> Terminator19/1
  Bus Selector7/1 -> dist_x/1, Human Follower model/5(this cars dist_x)  "<X>"
  Follower Vehicle1/4 -> Terminator13/1
  Follower Vehicle1/3 -> vel_y/1
  lead car vel_x/1 -> Human Follower model/2(lead cars vel_x)
  Follower Vehicle1/7 -> Terminator20/1
  Vector Concatenate4/1 -> Follower Vehicle1/1
  Follower Vehicle1/1 -> Bus Selector7/1
  Kinematic Steering3/1 -> Terminator16/1
  lead car dist_x/1 -> Human Follower model/4(lead cars dist_x)
  Bus Selector7/2 -> dist_y/1  "<Y>"
  sampling time/1 -> Human Follower model/6(sampling time)
  Kinematic Steering3/2 -> Vector Concatenate4/1
  stearing angle(rad)/1 -> Kinematic Steering3/1
  Kinematic Steering3/3 -> Vector Concatenate4/2
  Follower Vehicle1/2 -> Human Follower model/1(this cars vel), vel_x/1
  Coefficient of Friction: Dry1/1 -> Follower Vehicle1/3
  Reaction Time/1(v_out) -> Follower Vehicle1/2, Reaction Time/2(v_old)
  Human Follower model/1(cmd Vel) -> Reaction Time/1(v_new)

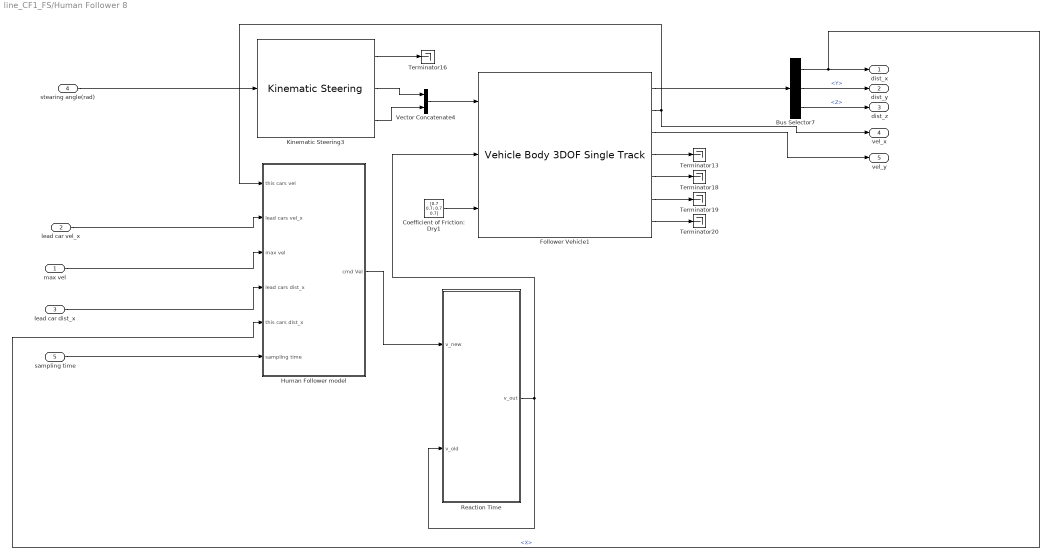
== system line_CF1_FS/Human Follower 8 ==
  max vel : Inport
  lead car vel_x : Inport  Port=2
  lead car dist_x : Inport  Port=3
  stearing angle(rad) : Inport  Port=4
  sampling time : Inport  Port=5
  Bus Selector7 : BusSelector  OutputSignals=InertFrm.Cg.Disp.X,InertFrm.Cg.Disp.Y,InertFrm.Cg.Disp.Z
  Coefficient of Friction: Dry1 : Constant  Value=[0.7 0.7; 0.7 0.7]
  Follower Vehicle1 : autolibshared/Vehicle Body 3DOF Single Track  trackMode=Dual  inputMode=External longitudinal velocity  frontSteerMode=on  rearSteerMode=off  windMode=off  muMode=on  extFMode=off  extMMode=off  aMode=2  NF=2  NR=2  m=2000  a=1.4  b=1.6  h=0.35  X_o=10  xdot_o=0  CalphaMode=off  sigmaMode=on  d=0  w=[1.4,1.4]  Cy_f=12e3  Cy_r=11e3  sigma_f=.1  sigma_r=.1  alpha_f_brk=[-.1 .1]  Cy_f_data=[-9e3 9e3]  alpha_r_brk=[-.1 .1]  Cy_r_data=[-9e3 9e3]  Y_o=0  ydot_o=0  Izz=4000  psi_o=0  r_o=0  Af=2  Cd=.3  Cl=.1  Cpm=.1  beta_w=[0:0.01:0.3]  Cs=[0:0.03:0.9]  Cym=[0:0.01:0.3]  Pabs=101325  Tair=273  g=9.81  mu=1  xdot_tol=.01  Fznom=5000  Fxtire_sat=7e4  Fytire_sat=7e4  longOff=0  latOff=0  vertOff=0
      settings: SourceProductName=Powertrain Blockset  SourceProductBaseCode=PW
  Human Follower model : Subsystem
  Kinematic Steering3 : vehdynlibsteering/Kinematic Steering  StrgType=Rack and pinion  StrgRatioType=Constant  Loc=Front  NrmlFctr=0.01  TrckWdth=1  WhlBase=1.524  Db=0  StrgRng=1.25*pi  StrgAngBpts="[-6.2832   -5.0265   -3.7699   -2.5133   -1.2566         0    1.2566    2.5133    3.7699    5.0265    6.2832]"  StrgRatioTbl=|  StrgRatio=100  StrgArmLngth=0.1  RckCsLngth=0.5  TieRodLngth=0.248  D=0.2  PnnRadius=0.0057  PnnRadiusTbl="[0.0055    0.0055    0.0056    0.0057    0.0058    0.0057    0.0057    0.0057    0.0056    0.0055    0.0055]"  RodLngth=0.1  ParaArmLngth=0.9  aMode=2
      | [13.5000   13.3750   13.2500   13.1250   13.0000   13.0000   13.0000   13.1250   13.2500   13.3750   13.5000
      | ]
      settings: SourceProductName=Vehicle Dynamics Blockset
  Reaction Time : Subsystem
  Terminator{13,16,18..20} (5 alike) : Terminator
  Vector Concatenate4 : Concatenate
  dist_x : Outport
  dist_y : Outport  Port=2
  dist_z : Outport  Port=3
  vel_x : Outport  Port=4
  vel_y : Outport  Port=5
  wires:
  Bus Selector7/3 -> dist_z/1  "<Z>"
  Follower Vehicle1/5 -> Terminator18/1
  max vel/1 -> Human Follower model/3(max vel)
  Follower Vehicle1/6 -> Terminator19/1
  Bus Selector7/1 -> dist_x/1, Human Follower model/5(this cars dist_x)  "<X>"
  Follower Vehicle1/4 -> Terminator13/1
  Follower Vehicle1/3 -> vel_y/1
  lead car vel_x/1 -> Human Follower model/2(lead cars vel_x)
  Follower Vehicle1/7 -> Terminator20/1
  Vector Concatenate4/1 -> Follower Vehicle1/1
  Follower Vehicle1/1 -> Bus Selector7/1
  Kinematic Steering3/1 -> Terminator16/1
  lead car dist_x/1 -> Human Follower model/4(lead cars dist_x)
  Bus Selector7/2 -> dist_y/1  "<Y>"
  sampling time/1 -> Human Follower model/6(sampling time)
  Kinematic Steering3/2 -> Vector Concatenate4/1
  stearing angle(rad)/1 -> Kinematic Steering3/1
  Kinematic Steering3/3 -> Vector Concatenate4/2
  Follower Vehicle1/2 -> Human Follower model/1(this cars vel), vel_x/1
  Coefficient of Friction: Dry1/1 -> Follower Vehicle1/3
  Reaction Time/1(v_out) -> Follower Vehicle1/2, Reaction Time/2(v_old)
  Human Follower model/1(cmd Vel) -> Reaction Time/1(v_new)

== system line_CF1_FS/FollowerStopper Controller/Dead Man's Switch ==
  note: The timeout value, and step size, are critical to set correctly here.
  IsNew : Inport
  value : Inport  Port=2
  Simulate step size : Constant  Value=stepSize
  Timeout in seconds : Constant  Value=timeout
  timeout set to 0 output : MATLAB Function  TreatAsAtomicUnit=on
  safeValue : Outport  InitialOutput=[0]
  timedOut : Outport  Port=2  InitialOutput=[0]
  wires:
  Simulate step size/1 -> timeout set to 0 output/4(stepSize)
  timeout set to 0 output/2(timedOut) -> timedOut/1
  Timeout in seconds/1 -> timeout set to 0 output/3(timeout)
  value/1 -> timeout set to 0 output/2(value)
  timeout set to 0 output/1(safeValue) -> safeValue/1
  IsNew/1 -> timeout set to 0 output/1(isNew)

== system line_CF1_FS/FollowerStopper Controller/Follower Stopper Controller ==
  note: \alpha_{1,2,3}
  note: \omega_3
  note: \omega_1
  note: Relative distance
  note: Reference Velocity
  note: Velocity of AV
  note: Relative velocity of
      | AV wrt lead vehicle
  note: Note that Benni's
      | controller uses dU
      | for relative
      | velocity
  r : Inport
  deltaV : Inport  Port=2
  deltaX : Inport  Port=3
  vel : Inport  Port=4
  decel : Inport  Port=5
  dx_min : Inport  Port=6
  dx_activate : Inport  Port=7
  MATLAB Function : MATLAB Function  TreatAsAtomicUnit=on
  Scope1 : Scope  NumInputPorts=2
  u_cmd : Outport
  wires:
  r/1 -> MATLAB Function/1(r)
  dx_activate/1 -> MATLAB Function/6(dx_activate)
  decel/1 -> MATLAB Function/7(decel)
  dx_min/1 -> MATLAB Function/5(dx_min)
  vel/1 -> MATLAB Function/4(v_AV)
  MATLAB Function/1(u_cmd) -> u_cmd/1
  deltaV/1 -> Scope1/1, MATLAB Function/3(dv)
  deltaX/1 -> Scope1/2, MATLAB Function/2(dx)

== system line_CF1_FS/FollowerStopper Controller/Parameters ==
  note: \alpha_{1,2,3}
  note: \omega_1
  note: \omega_3
  Get Parameter1 : robotlib/Get Parameter  ParameterSource=Specify your own  ParameterName=/dx_min  ParameterType=double  ParameterMaxArrayLength=16  ParameterInitialValue=4.5  SampleTime=-1  ShowErrorCodeOutput=off  ModelName=line_CF1_FS  BlockId=ParamGet_line_CF1_FS_61
      settings: SourceProductName=Robotics System Toolbox  SourceProductBaseCode=RO
  Get Parameter2 : robotlib/Get Parameter  ParameterSource=Specify your own  ParameterName=/dx_activate  ParameterType=double  ParameterMaxArrayLength=16  ParameterInitialValue=6.0  SampleTime=-1  ShowErrorCodeOutput=off  ModelName=line_CF1_FS  BlockId=ParamGet_line_CF1_FS_62
      settings: SourceProductName=Robotics System Toolbox  SourceProductBaseCode=RO
  decel : Constant  Value=[1.5 1.0 0.5]  OutDataTypeStr=double  SampleTime=-1
  alpha : Outport
  omega_1 : Outport  Port=2
  omega_3 : Outport  Port=3
  wires:
  decel/1 -> alpha/1
  Get Parameter1/1 -> omega_1/1
  Get Parameter2/1 -> omega_3/1

== system line_CF1_FS/FollowerStopper Controller/smoothUp Parameters ==
  In1 : Inport
  Terminator : Terminator
  max_accel1 : Constant  Value=1.5
  max_decel1 : Constant  Value=-1.5
  reference_vel1 : Constant  Value=3.748509500812156
  reference_vel : Outport
  max_accel : Outport  Port=2
  max_decel : Outport  Port=3
  wires:
  In1/1 -> Terminator/1
  reference_vel1/1 -> reference_vel/1
  max_accel1/1 -> max_accel/1
  max_decel1/1 -> max_decel/1

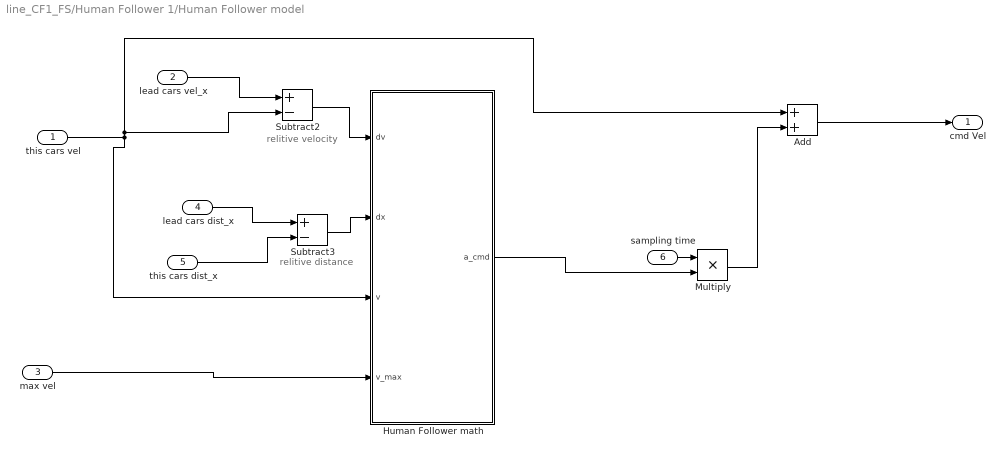
== system line_CF1_FS/Human Follower 1/Human Follower model ==
  note: relitive distance
  note: relitive velocity
  this cars vel : Inport
  lead cars vel_x : Inport  Port=2
  max vel : Inport  Port=3
  lead cars dist_x : Inport  Port=4
  this cars dist_x : Inport  Port=5
  sampling time : Inport  Port=6
  Add : Sum
  Human Follower math : Subsystem
  Multiply : Product
  Subtract2 : Sum  Inputs=+-
  Subtract3 : Sum  Inputs=+-
  cmd Vel : Outport
  wires:
  Add/1 -> cmd Vel/1
  lead cars dist_x/1 -> Subtract3/1
  this cars vel/1 -> Human Follower math/3(v), Add/1, Subtract2/2
  Human Follower math/1(a_cmd) -> Multiply/2
  Subtract3/1 -> Human Follower math/2(dx)
  Multiply/1 -> Add/2
  this cars dist_x/1 -> Subtract3/2
  Subtract2/1 -> Human Follower math/1(dv)
  max vel/1 -> Human Follower math/4(v_max)
  lead cars vel_x/1 -> Subtract2/1
  sampling time/1 -> Multiply/1

== system line_CF1_FS/Human Follower 1/Reaction Time ==
  v_new : Inport
  v_old : Inport  Port=2
  Delay : Delay  DelayLength=3  InitialConditionSource=Input port
      settings: InputPortMap=u0,p4
  If Action Subsystem3 : Subsystem  TreatAsAtomicUnit=on
  If Action Subsystem5 : Subsystem  TreatAsAtomicUnit=on
  If2 : If  NumInputs=2  IfExpression=u2 ~= u1
  Merge1 : Merge
  v_out : Outport
  wires:
  If Action Subsystem5/1(Out1) -> Merge1/2
  If2/1 -> If Action Subsystem3/Action
  If2/2 -> If Action Subsystem5/Action
  If Action Subsystem3/1(Out1) -> Merge1/1
  v_new/1 -> If2/1, If Action Subsystem3/1(In1)
  Merge1/1 -> Delay/1
  Delay/1 -> v_out/1
  v_old/1 -> If2/2, Delay/2, If Action Subsystem5/1(In1)

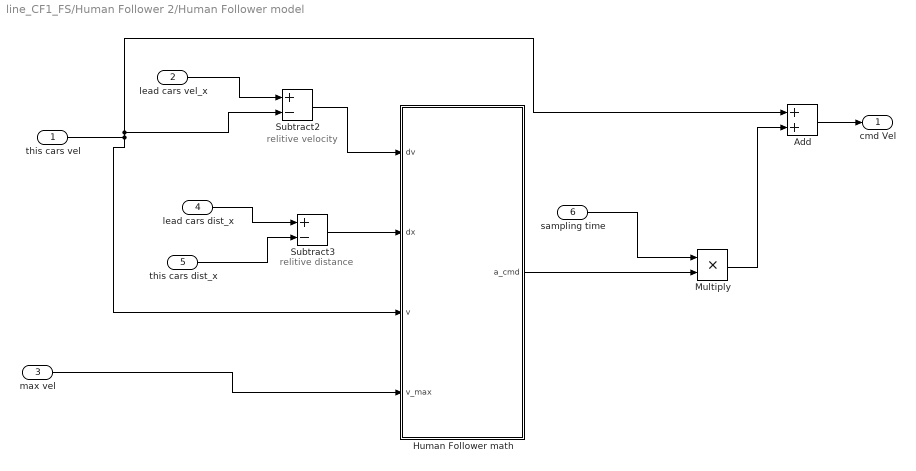
== system line_CF1_FS/Human Follower 2/Human Follower model ==
  note: relitive distance
  note: relitive velocity
  this cars vel : Inport
  lead cars vel_x : Inport  Port=2
  max vel : Inport  Port=3
  lead cars dist_x : Inport  Port=4
  this cars dist_x : Inport  Port=5
  sampling time : Inport  Port=6
  Add : Sum
  Human Follower math : Subsystem
  Multiply : Product
  Subtract2 : Sum  Inputs=+-
  Subtract3 : Sum  Inputs=+-
  cmd Vel : Outport
  wires:
  Add/1 -> cmd Vel/1
  lead cars dist_x/1 -> Subtract3/1
  this cars vel/1 -> Human Follower math/3(v), Add/1, Subtract2/2
  Human Follower math/1(a_cmd) -> Multiply/2
  Subtract3/1 -> Human Follower math/2(dx)
  Multiply/1 -> Add/2
  this cars dist_x/1 -> Subtract3/2
  Subtract2/1 -> Human Follower math/1(dv)
  max vel/1 -> Human Follower math/4(v_max)
  sampling time/1 -> Multiply/1
  lead cars vel_x/1 -> Subtract2/1

== system line_CF1_FS/Human Follower 2/Reaction Time ==
  v_new : Inport
  v_old : Inport  Port=2
  Delay : Delay  DelayLength=3  InitialConditionSource=Input port  InitialCondition=0
      settings: InputPortMap=u0,p4
  If Action Subsystem3 : Subsystem  TreatAsAtomicUnit=on
  If Action Subsystem5 : Subsystem  TreatAsAtomicUnit=on
  If2 : If  NumInputs=2  IfExpression=u2 ~= u1
  Merge1 : Merge
  v_out : Outport
  wires:
  If Action Subsystem5/1(Out1) -> Merge1/2
  If2/1 -> If Action Subsystem3/Action
  If2/2 -> If Action Subsystem5/Action
  If Action Subsystem3/1(Out1) -> Merge1/1
  v_new/1 -> If2/1, If Action Subsystem3/1(In1)
  Merge1/1 -> Delay/1
  Delay/1 -> v_out/1
  v_old/1 -> If2/2, Delay/2, If Action Subsystem5/1(In1)

== system line_CF1_FS/Human Follower 3/Human Follower model ==
  note: relitive distance
  note: relitive velocity
  this cars vel : Inport
  lead cars vel_x : Inport  Port=2
  max vel : Inport  Port=3
  lead cars dist_x : Inport  Port=4
  this cars dist_x : Inport  Port=5
  sampling time : Inport  Port=6
  Add : Sum
  Human Follower math : Subsystem
  Multiply : Product
  Subtract2 : Sum  Inputs=+-
  Subtract3 : Sum  Inputs=+-
  cmd Vel : Outport
  wires:
  Add/1 -> cmd Vel/1
  lead cars dist_x/1 -> Subtract3/1
  this cars vel/1 -> Human Follower math/3(v), Add/1, Subtract2/2
  Human Follower math/1(a_cmd) -> Multiply/2
  Subtract3/1 -> Human Follower math/2(dx)
  Multiply/1 -> Add/2
  this cars dist_x/1 -> Subtract3/2
  Subtract2/1 -> Human Follower math/1(dv)
  max vel/1 -> Human Follower math/4(v_max)
  sampling time/1 -> Multiply/1
  lead cars vel_x/1 -> Subtract2/1

== system line_CF1_FS/Human Follower 3/Reaction Time ==
  v_new : Inport
  v_old : Inport  Port=2
  Delay : Delay  DelayLength=3  InitialConditionSource=Input port
      settings: InputPortMap=u0,p4
  If Action Subsystem3 : Subsystem  TreatAsAtomicUnit=on
  If Action Subsystem5 : Subsystem  TreatAsAtomicUnit=on
  If2 : If  NumInputs=2  IfExpression=u2 ~= u1
  Merge1 : Merge
  v_out : Outport
  wires:
  If Action Subsystem5/1(Out1) -> Merge1/2
  If2/1 -> If Action Subsystem3/Action
  If2/2 -> If Action Subsystem5/Action
  If Action Subsystem3/1(Out1) -> Merge1/1
  v_new/1 -> If2/1, If Action Subsystem3/1(In1)
  Merge1/1 -> Delay/1
  Delay/1 -> v_out/1
  v_old/1 -> If2/2, Delay/2, If Action Subsystem5/1(In1)

== system line_CF1_FS/Human Follower 4/Human Follower model ==
  note: relitive distance
  note: relitive velocity
  this cars vel : Inport
  lead cars vel_x : Inport  Port=2
  max vel : Inport  Port=3
  lead cars dist_x : Inport  Port=4
  this cars dist_x : Inport  Port=5
  sampling time : Inport  Port=6
  Add : Sum
  Human Follower math : Subsystem
  Multiply : Product
  Subtract2 : Sum  Inputs=+-
  Subtract3 : Sum  Inputs=+-
  cmd Vel : Outport
  wires:
  Add/1 -> cmd Vel/1
  lead cars dist_x/1 -> Subtract3/1
  this cars vel/1 -> Human Follower math/3(v), Add/1, Subtract2/2
  Human Follower math/1(a_cmd) -> Multiply/2
  Subtract3/1 -> Human Follower math/2(dx)
  Multiply/1 -> Add/2
  this cars dist_x/1 -> Subtract3/2
  Subtract2/1 -> Human Follower math/1(dv)
  max vel/1 -> Human Follower math/4(v_max)
  sampling time/1 -> Multiply/1
  lead cars vel_x/1 -> Subtract2/1
